simulink model "mdl_VD_dt7dofModelWithSteeringControl"  (R2019b)
settings: Solver=ode4  StartTime=0.0  StopTime=50  FixedStep=deltaT  RelTol=1e-4  EnableMultiTasking=on
values from neighbouring files (symbols this model uses):
  deltaT = 0.01    [script_test_mdl_VD_dt7dofModel.m]    (also in script_test_mdl_VD_dt7dofModelFriction.m; script_test_mdl_VD_dtNormalForce.m; script_test_mdl_VD_dtSlipAngle.m; script_test_mdl_VD_dtWheelSlip.m)
  friction_coefficient = [0.9, 0.9, 0.9, 0.9]    [script_test_mdl_VD_dt7dofModel.m]    (also in script_test_mdl_VD_dt7dofModelFriction.m)
  inputTrajectory = swervedVehicleTrajectory    [script_simulateFrictionUtilization.m]
  wheel_torque = [0, 0, 3, 3]    [script_test_mdl_VD_dt7dofModel.m]    (also in script_test_mdl_VD_dt7dofModelFriction.m)
undefined symbols (not defined in the file or in its folder): controller, initial, road_properties, vdParam, vehicle
libraries: simulink x7
(part 2 of 2)

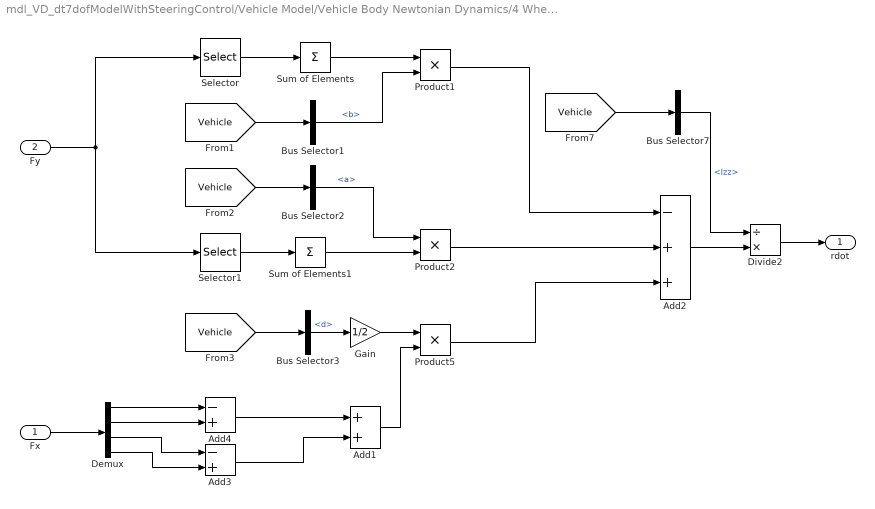
== system mdl_VD_dt7dofModelWithSteeringControl/Vehicle Model/Vehicle Body Newtonian Dynamics/4 Wheel rdot ==
  Fx : Inport
  Fy : Inport  Port=2
  Add1 : Sum
  Add2 : Sum  Inputs=-++
  Add3 : Sum  Inputs=-+
  Add4 : Sum  Inputs=-+
  Bus Selector1 : BusSelector  OutputSignals=b
  Bus Selector2 : BusSelector  OutputSignals=a
  Bus Selector3 : BusSelector  OutputSignals=d
  Bus Selector7 : BusSelector  OutputSignals=Izz
  Demux : Demux
  Divide2 : Product  Inputs=/*
  Gain : Gain  Gain=1/2
  Product1 : Product  RndMeth=Zero
  Product2 : Product  RndMeth=Zero
  Product5 : Product  RndMeth=Zero
  Selector : Selector  InputPortWidth=4  IndexOptions=Index vector (dialog)  Indices=[3 4]  OutputSizes=1
  Selector1 : Selector  InputPortWidth=4  IndexOptions=Index vector (dialog)  Indices=[1 2]  OutputSizes=1
  Sum of Elements : Sum  Inputs=+
  Sum of Elements1 : Sum  Inputs=+
  rdot : Outport
  wires:
  Fy/1 -> Selector/1, Selector1/1
  Divide2/1 -> rdot/1
  Bus Selector7/1 -> Divide2/1  "<Izz>"
  Add2/1 -> Divide2/2
  [Vehicle] -> Bus Selector7/1
  [Vehicle] -> Bus Selector1/1
  Selector/1 -> Sum of Elements/1
  Selector1/1 -> Sum of Elements1/1
  Sum of Elements/1 -> Product1/1
  Bus Selector1/1 -> Product1/2  "<b>"
  Product1/1 -> Add2/1
  Fx/1 -> Demux/1
  [Vehicle] -> Bus Selector2/1
  Product2/1 -> Add2/2
  Bus Selector2/1 -> Product2/1  "<a>"
  Sum of Elements1/1 -> Product2/2
  Demux/3 -> Add3/1
  Demux/4 -> Add3/2
  Demux/1 -> Add4/1
  Demux/2 -> Add4/2
  Add4/1 -> Add1/1
  [Vehicle] -> Bus Selector3/1
  Add1/1 -> Product5/2
  Bus Selector3/1 -> Gain/1  "<d>"
  Gain/1 -> Product5/1
  Product5/1 -> Add2/3
  Add3/1 -> Add1/2

== system mdl_VD_dt7dofModelWithSteeringControl/Vehicle Model/Vehicle Body Newtonian Dynamics/Wheel to Body Transform ==
  note: ISO Coordinate Transform
  Fy_Wheel : Inport
  Fx_Wheel : Inport  Port=2
  delta : Inport  Port=3
  Add : Sum
  Cos1 : Trigonometry
  Cos2 : Trigonometry  Operator=cos
  Cos8 : Trigonometry  Operator=cos
  Cos9 : Trigonometry
  Fx_Wheel1 : InportShadow  Port=2
  Fy_Wheel1 : InportShadow
  Product{4..7} (4 alike) : Product
  Subtract : Sum  Inputs=+-
  Fx_Body : Outport
  Fy_Body : Outport  Port=2
  wires:
  Subtract/1 -> Fx_Body/1
  delta/1 -> Cos8/1, Cos9/1, Cos2/1, Cos1/1
  Cos8/1 -> Product4/1
  Cos9/1 -> Product5/1
  Cos1/1 -> Product6/1
  Cos2/1 -> Product7/1
  Fx_Wheel1/1 -> Product6/2
  Fy_Wheel1/1 -> Product7/2
  Fy_Wheel/1 -> Product5/2
  Fx_Wheel/1 -> Product4/2
  Product4/1 -> Subtract/1
  Product5/1 -> Subtract/2
  Product6/1 -> Add/1
  Product7/1 -> Add/2
  Add/1 -> Fy_Body/1

== system mdl_VD_dt7dofModelWithSteeringControl/Friction Estimation/Normal Force/Normal Force Static/Lateral Transfer_Banking ==
  Road Geometry : Inport
  Bus Selector : BusSelector  OutputSignals=banking angle
  Bus Selector4 : BusSelector  OutputSignals=b,L,a
  Bus Selector6 : BusSelector  OutputSignals=m,h_cg,d
  Divide3 : Product  Inputs=*/
  Divide4 : Product  Inputs=/*
  Product1 : Product  RndMeth=Zero
  Product2 : Product  RndMeth=Zero
  Product4 : Product  Inputs=*/  RndMeth=Zero
  Product5 : Product  Inputs=3  RndMeth=Zero
  Product6 : Product  RndMeth=Zero
  Trigonometric Function2 : Trigonometry
  g : Constant  Value=9.81
  Lateral Transfer Front : Outport
  Lateral Transfer Rear : Outport  Port=2
  wires:
  g/1 -> Product5/2
  Road Geometry/1 -> Bus Selector/1
  Trigonometric Function2/1 -> Product5/1
  Bus Selector/1 -> Trigonometric Function2/1  "<banking angle>"
  Divide4/1 -> Product1/1
  Bus Selector6/1 -> Product5/3  "<m>"
  Product2/1 -> Lateral Transfer Front/1
  Product4/1 -> Product6/2
  [Vehicle] -> Bus Selector4/1
  Product6/1 -> Product2/1, Product1/2
  Bus Selector6/2 -> Product4/1  "<h_cg>"
  Bus Selector4/3 -> Divide4/2  "<a>"
  Divide3/1 -> Product2/2
  [Vehicle] -> Bus Selector6/1
  Bus Selector6/3 -> Product4/2  "<d>"
  Bus Selector4/2 -> Divide3/2, Divide4/1  "<L>"
  Product1/1 -> Lateral Transfer Rear/1
  Product5/1 -> Product6/1
  Bus Selector4/1 -> Divide3/1  "<b>"

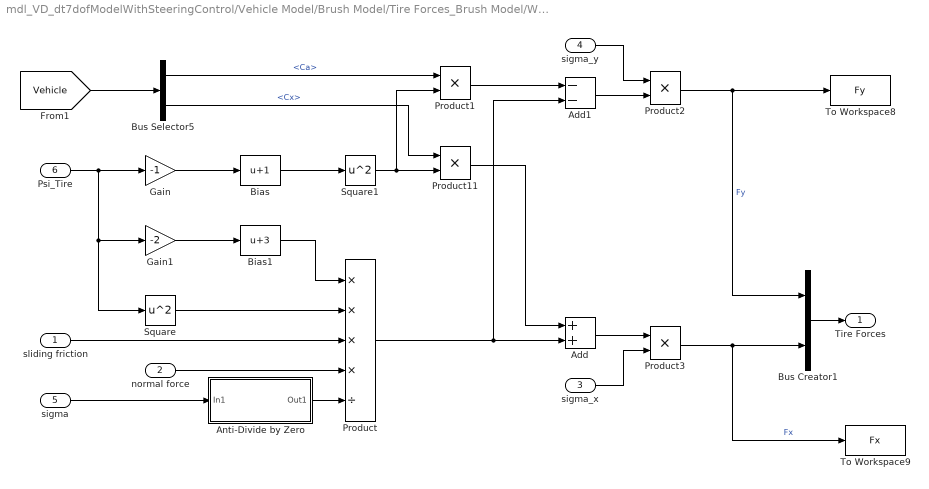
== system mdl_VD_dt7dofModelWithSteeringControl/Vehicle Model/Brush Model/Tire Forces_Brush Model/Wheel Forces ==
  sliding friction : Inport
  normal force : Inport  Port=2
  sigma_x : Inport  Port=3
  sigma_y : Inport  Port=4
  sigma : Inport  Port=5
  Psi_Tire : Inport  Port=6
  Add : Sum
  Add1 : Sum  Inputs=--
  Anti-Divide by Zero : Subsystem
  Bias : Bias  Bias=1
  Bias1 : Bias  Bias=3
  Bus Creator1 : BusCreator  Inputs=2
  Bus Selector5 : BusSelector  OutputSignals=Ca,Cx
  Gain : Gain  Gain=-1
  Gain1 : Gain  Gain=-2
  Product : Product  Inputs=****/
  Product{1..3,11} (4 alike) : Product  RndMeth=Zero
  Square : Math  Operator=square  SignedPower=off  SaturateOnIntegerOverflow=on
  Square1 : Math  Operator=square  SignedPower=off  SaturateOnIntegerOverflow=on
  To Workspace8 : ToWorkspace  VariableName=Fy  SampleTime=-1
  To Workspace9 : ToWorkspace  VariableName=Fx  SampleTime=-1
  Tire Forces : Outport
  wires:
  Product/1 -> Add1/2, Add/2
  Bus Selector5/2 -> Product11/1  "<Cx>"
  [Vehicle] -> Bus Selector5/1
  Gain/1 -> Bias/1
  Gain1/1 -> Bias1/1
  Bias/1 -> Square1/1
  Psi_Tire/1 -> Square/1, Gain1/1, Gain/1
  Square/1 -> Product/2
  Bias1/1 -> Product/1
  sliding friction/1 -> Product/3
  normal force/1 -> Product/4
  sigma/1 -> Anti-Divide by Zero/1(In1)
  Square1/1 -> Product1/2, Product11/2
  Product11/1 -> Add/1
  Bus Selector5/1 -> Product1/1  "<Ca>"
  Product1/1 -> Add1/1
  Add1/1 -> Product2/2
  sigma_y/1 -> Product2/1
  sigma_x/1 -> Product3/2
  Add/1 -> Product3/1
  Bus Creator1/1 -> Tire Forces/1
  Product2/1 -> Bus Creator1/1, To Workspace8/1  "Fy"
  Product3/1 -> To Workspace9/1, Bus Creator1/2  "Fx"
  Anti-Divide by Zero/1(Out1) -> Product/5

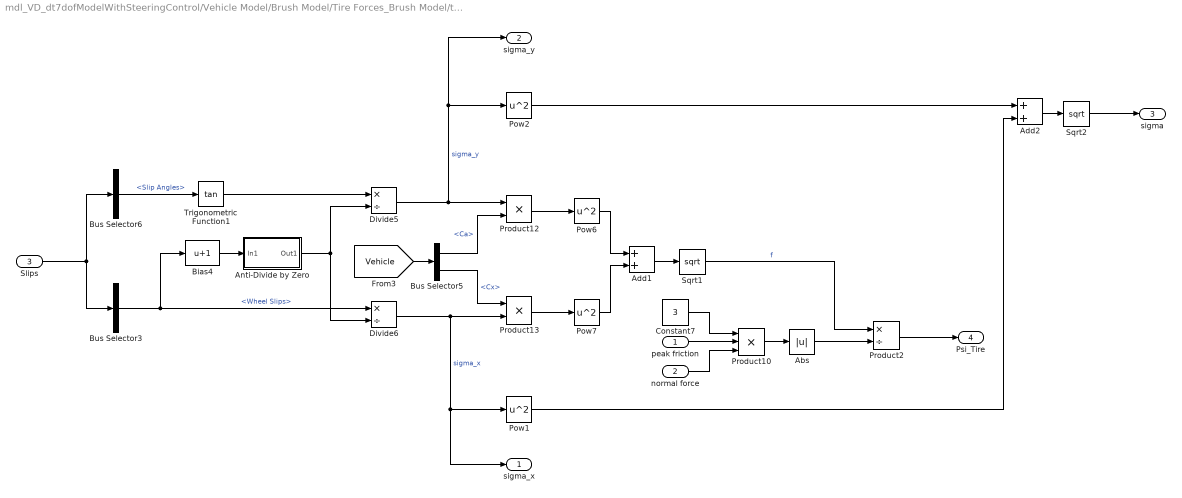
== system mdl_VD_dt7dofModelWithSteeringControl/Vehicle Model/Brush Model/Tire Forces_Brush Model/tire slip ==
  peak friction : Inport
  normal force : Inport  Port=2
  Slips : Inport  Port=3
  Abs : Abs
  Add1 : Sum
  Add2 : Sum
  Anti-Divide by Zero : Subsystem
  Bias4 : Bias  Bias=1
  Bus Selector3 : BusSelector  OutputSignals=Wheel Slips
  Bus Selector5 : BusSelector  OutputSignals=Ca,Cx
  Bus Selector6 : BusSelector  OutputSignals=Slip Angles
  Constant7 : Constant  Value=3
  Divide5 : Product  Inputs=*/
  Divide6 : Product  Inputs=*/
  Pow{1..2,6..7} (4 alike) : Math  Operator=square  SaturateOnIntegerOverflow=on
  Product10 : Product  Inputs=3  RndMeth=Zero
  Product12 : Product  RndMeth=Zero
  Product13 : Product  RndMeth=Zero
  Product2 : Product  Inputs=*/  RndMeth=Zero
  Sqrt1 : Sqrt  SaturateOnIntegerOverflow=on
  Sqrt2 : Sqrt  SaturateOnIntegerOverflow=on
  Trigonometric Function1 : Trigonometry  Operator=tan
  sigma_x : Outport
  sigma_y : Outport  Port=2
  sigma : Outport  Port=3
  Psi_Tire : Outport  Port=4
  wires:
  Sqrt2/1 -> sigma/1
  Pow7/1 -> Add1/2
  Slips/1 -> Bus Selector6/1, Bus Selector3/1
  normal force/1 -> Product10/3
  Product12/1 -> Pow6/1
  Sqrt1/1 -> Product2/1  "f"
  Bus Selector5/2 -> Product13/1  "<Cx>"
  Pow2/1 -> Add2/1
  peak friction/1 -> Product10/2
  Product10/1 -> Abs/1
  Anti-Divide by Zero/1(Out1) -> Divide6/2, Divide5/2
  Constant7/1 -> Product10/1
  Pow1/1 -> Add2/2
  Trigonometric Function1/1 -> Divide5/1
  Add2/1 -> Sqrt2/1
  Divide6/1 -> sigma_x/1, Pow1/1, Product13/2  "sigma_x"
  Product13/1 -> Pow7/1
  Bus Selector3/1 -> Divide6/1, Bias4/1  "<Wheel Slips>"
  Pow6/1 -> Add1/1
  Divide5/1 -> sigma_y/1, Pow2/1, Product12/1  "sigma_y"
  Product2/1 -> Psi_Tire/1
  [Vehicle] -> Bus Selector5/1
  Bus Selector6/1 -> Trigonometric Function1/1  "<Slip Angles>"
  Bias4/1 -> Anti-Divide by Zero/1(In1)
  Bus Selector5/1 -> Product12/2  "<Ca>"
  Add1/1 -> Sqrt1/1
  Abs/1 -> Product2/2

== system mdl_VD_dt7dofModelWithSteeringControl/Vehicle Model/Normal Force/Normal Force Static/Lateral Transfer_Banking ==
  Road Geometry : Inport
  Bus Selector : BusSelector  OutputSignals=road geometry.banking angle
  Bus Selector4 : BusSelector  OutputSignals=b,L,a
  Bus Selector6 : BusSelector  OutputSignals=m,h_cg,d
  Divide3 : Product  Inputs=*/
  Divide4 : Product  Inputs=/*
  Product1 : Product  RndMeth=Zero
  Product2 : Product  RndMeth=Zero
  Product4 : Product  Inputs=*/  RndMeth=Zero
  Product5 : Product  Inputs=3  RndMeth=Zero
  Product6 : Product  RndMeth=Zero
  Trigonometric Function2 : Trigonometry
  g : Constant  Value=9.81
  Lateral Transfer Front : Outport
  Lateral Transfer Rear : Outport  Port=2
  wires:
  g/1 -> Product5/2
  Road Geometry/1 -> Bus Selector/1
  Trigonometric Function2/1 -> Product5/1
  Bus Selector/1 -> Trigonometric Function2/1  "<banking angle>"
  Divide4/1 -> Product1/1
  Bus Selector6/1 -> Product5/3  "<m>"
  Product2/1 -> Lateral Transfer Front/1
  Product4/1 -> Product6/2
  [Vehicle] -> Bus Selector4/1
  Product6/1 -> Product2/1, Product1/2
  Bus Selector6/2 -> Product4/1  "<h_cg>"
  Bus Selector4/3 -> Divide4/2  "<a>"
  Divide3/1 -> Product2/2
  [Vehicle] -> Bus Selector6/1
  Bus Selector6/3 -> Product4/2  "<d>"
  Bus Selector4/2 -> Divide3/2, Divide4/1  "<L>"
  Product1/1 -> Lateral Transfer Rear/1
  Product5/1 -> Product6/1
  Bus Selector4/1 -> Divide3/1  "<b>"

== system mdl_VD_dt7dofModelWithSteeringControl/Vehicle Model/Slips/Wheel Slip Ratio/Wheel Slip ==
  note: κ>0, acceleration→ positive Fx
      | κ<0, braking → negative Fx
  Vx_tire : Inport
  Speeds : Inport  Port=2
  Anti-Divide by Zero : Subsystem
  Bus Selector2 : BusSelector  OutputSignals=Re
  Bus Selector4 : BusSelector  OutputSignals=omega
  Divide2 : Product  Inputs=/*
  Product2 : Product  RndMeth=Zero
  Saturation : Saturate  UpperLimit=1  LowerLimit=-1  ZeroCross=off
  Subtract2 : Sum  Inputs=-+
  Switch1 : Switch  Criteria=u2 > Threshold  ZeroCross=off  SaturateOnIntegerOverflow=on
  zero Wheel Slip : Constant  Value=[0 0 0 0]
  Wheel Slips : Outport
  wires:
  Subtract2/1 -> Divide2/2
  Anti-Divide by Zero/1(Out1) -> Divide2/1
  zero Wheel Slip/1 -> Switch1/3
  Vx_tire/1 -> Anti-Divide by Zero/1(In1), Subtract2/1, Switch1/2
  Bus Selector2/1 -> Product2/2  "<Re>"
  [Vehicle] -> Bus Selector2/1
  Divide2/1 -> Switch1/1
  Switch1/1 -> Saturation/1
  Product2/1 -> Subtract2/2
  Saturation/1 -> Wheel Slips/1  "Wheel Slips"
  Bus Selector4/1 -> Product2/1  "<omega>"
  Speeds/1 -> Bus Selector4/1

== system mdl_VD_dt7dofModelWithSteeringControl/Vehicle Model/Slips/Wheel Slip Ratio/vehicle2tire ==
  note: ISO Coordinate System
  delta : Inport
  Speeds : Inport  Port=2
  Add : Sum
  Add1 : Sum
  Add2 : Sum
  Bus Selector1 : BusSelector  OutputSignals=d,a,b
  Bus Selector4 : BusSelector  OutputSignals=r,Vy
  Bus Selector7 : BusSelector  OutputSignals=Vx
  Cos : Trigonometry  Operator=cos
  Gain : Gain  Gain=1/2
  Mux1 : Mux
  Mux2 : Mux
  Product{,1..4} (5 alike) : Product  RndMeth=Zero
  Sin : Trigonometry
  Speeds1 : InportShadow  Port=2
  Subtract : Sum  Inputs=-+
  Subtract3 : Sum  Inputs=+-
  Vx_tire : Outport
  wires:
  Speeds1/1 -> Bus Selector7/1
  Bus Selector4/1 -> Product3/2, Product1/2, Product/2  "<r>"
  Bus Selector1/2 -> Product1/1  "<a>"
  Product3/1 -> Subtract3/2, Add1/2
  Bus Selector7/1 -> Add1/1, Subtract3/1  "<Vx>"
  Product/1 -> Subtract/1
  Bus Selector4/2 -> Add/2, Subtract/2  "<Vy>"
  [Vehicle] -> Bus Selector1/1
  Product1/1 -> Add/1
  Add/1 -> Mux1/1, Mux1/2  "Vy+ar"
  Mux2/1 -> Product2/1
  Mux1/1 -> Product4/2
  Bus Selector1/3 -> Product/1  "<b>"
  Gain/1 -> Product3/1
  Speeds/1 -> Bus Selector4/1
  Subtract/1 -> Mux1/4, Mux1/3  "Vy-br"
  Bus Selector1/1 -> Gain/1  "<d>"
  Subtract3/1 -> Mux2/1, Mux2/3  "Vx-dr/2"
  Add1/1 -> Mux2/4, Mux2/2  "Vx+dr/2"
  Product2/1 -> Add2/1
  Add2/1 -> Vx_tire/1
  delta/1 -> Cos/1, Sin/1
  Cos/1 -> Product2/2
  Sin/1 -> Product4/1
  Product4/1 -> Add2/2

== system mdl_VD_dt7dofModelWithSteeringControl/Vehicle Model/Brush Model/Tire Forces_Brush Model/Wheel Forces/Anti-Divide by Zero ==
  In1 : Inport
  Add : Sum
  Compare To Zero : simulink/Logic and Bit Operations/Compare To Zero  relop===  OutDataTypeStr=boolean
  Constant : Constant  Value=eps
  Product : Product
  Out1 : Outport
  wires:
  Add/1 -> Out1/1
  Compare To Zero/1 -> Product/1
  Constant/1 -> Product/2
  Product/1 -> Add/2
  In1/1 -> Compare To Zero/1, Add/1

== system mdl_VD_dt7dofModelWithSteeringControl/Vehicle Model/Brush Model/Tire Forces_Brush Model/tire slip/Anti-Divide by Zero ==
  In1 : Inport
  Add : Sum
  Compare To Zero : simulink/Logic and Bit Operations/Compare To Zero  relop===  OutDataTypeStr=boolean
  Constant : Constant  Value=eps
  Product : Product
  Out1 : Outport
  wires:
  Add/1 -> Out1/1
  Compare To Zero/1 -> Product/1
  Constant/1 -> Product/2
  Product/1 -> Add/2
  In1/1 -> Compare To Zero/1, Add/1

== system mdl_VD_dt7dofModelWithSteeringControl/Vehicle Model/Slips/Wheel Slip Ratio/Wheel Slip/Anti-Divide by Zero ==
  In1 : Inport
  Add : Sum
  Compare To Zero : simulink/Logic and Bit Operations/Compare To Zero  relop===  OutDataTypeStr=boolean
  Constant : Constant  Value=eps
  Product : Product
  Out1 : Outport
  wires:
  In1/1 -> Add/1, Compare To Zero/1
  Product/1 -> Add/2
  Constant/1 -> Product/2
  Compare To Zero/1 -> Product/1
  Add/1 -> Out1/1

== matlab function mdl_VD_dt7dofModelWithSteeringControl/Friction Estimation/Noise Models/GPS Noise Function ==
  settings: updateMethod=DISCRETE
  data: v_x input; v_x_out output; v_y input; r input; sampling_time input; v_y_out output; r_out output
function [v_x_out, v_y_out, r_out] = GPS_noise(v_x, v_y, r, sampling_time)

% v_x: velocity in X direction [m/s]
% v_y: velocity in Y direction [m/s]
% r: the yaw rate [rad/s]
% sample_rate: frequency at which velocities are being calculated [Hz]

% sensor specifications
sigma_x = 0.025;
sigma_y = 0.025;
sigma_theta = 0.009;

% simulate noisy measurements
v_x_out = v_x + normrnd(0,1.4142*sigma_x)*sampling_time;
v_y_out = v_y + normrnd(0,1.4142*sigma_y)*sampling_time;
r_out   = r + normrnd(0,1.4142*sigma_theta)*sampling_time;

end

== matlab function mdl_VD_dt7dofModelWithSteeringControl/Friction Estimation/Noise Models/IMU Noise Function ==
  settings: updateMethod=DISCRETE
  data: a_x input; a_x_out output; a_y input; sampling_time input; a_y_out output
function [a_x_out, a_y_out] = IMU_noise(a_x, a_y, sampling_time)

% a_x: accelaration in X direction [m/s^2]
% a_y: accelaration in Y direction [m/s^2]
% alpha: the yaw angular accelaration [rad/s^2]
% sample_rate: frequency at which velocities are being calculated [Hz]

% sensor specifications
sigma_x = 0.25;
sigma_y = 0.25;
% sigma_theta = 0.09;

% simulate noisy measurements
a_x_out = a_x + normrnd(0,2*sigma_x)*(sampling_time^2);
a_y_out = a_y + normrnd(0,2*sigma_y)*(sampling_time^2);
% alpha_out = alpha_in + normrnd(0,2*sigma_theta)*(sampling_time^2);

end
